simulink library "Ampere_Library"  (R2022b)
settings: Solver=FixedStepDiscrete  StartTime=0  StopTime=10.0  RelTol=1e-3  EnableMultiTasking=on
undefined symbols (not defined in the file or in its folder): A_INST_double, Dem_EventStatusType, ECU_AMBIENT_TEMPERATURE, SET_ECU_AMBIENT_TEMPERATURE, SlDemoSign, Std_ReturnType
libraries: simulink x13
(part 4 of 10)

== system Ampere_Library/User_Defined_Libraries/Logic_and_Bit_Operations ==
  note: Comparisons to value
  note: Detect changes for
      | booleans
  note: Detect changes for
      | all data types
  note: Logic & Bit Operations
  A_CompareToConstant : Subsystem  Tag=[LIB]  mask(A_CompareToConstant){relop===, Const=1, ZeroCross=off}
      mask prompts: relop "Operator:"; Const "Constant value:"; ZeroCross "Enable zero-crossing detection"
      mask help:
      | Output will be one when the signal less than or equal to a constant otherwise it will be zero.
      |
      | The "Operator" parameter can have the following values:
      |       1. "==" - Determine whether the input is equal to Constant.
      |       2. "~=" - Determine whether the input is not equal to Constant.
      |       3. "<"  - Determine whether the input is less than Constant.
      |       4. "<=" - Determine whether the input is less than or equal to Constant.
      |       5. ">"  - Determine whether the input is greater than Constant.
      |       6. ">=" - Determine whether the input is greater than or equal to Constant.
      |
      | Note:
      |       1. Input Datatype of the block must NOT be "Double" and "Single" when "==" or "~="  is used
      mask init:
      | %% Update internal relop block
      | set_param ([gcb,'/Compare'],'relop',relop, ...
      |     'ZeroCross', ZeroCross);
      settings: AttributesFormatString=%<MaskType>
      mask TypeOptions relop: == | ~= | < | <= | >= | >
      mask Callback ZeroCross:
      | % Update tag depending on the mask option Enable zero-crossing detection
      | if strcmp(get_param(gcb,'ZeroCross'),'on')
      |     % Display the SaturateOnOverflow parameter
      |     set_param(gcb, 'AttributesFormatString', sprintf('%%<MaskType>\nzero-crossing = on'));
      | else
      |     % Do not display the SaturateOnOverflow parameter
      |     set_param(gcb, 'AttributesFormatString', sprintf('%%<MaskType>\n'));
      | end
      mask Display:
      | %% Display info on the icon
      | fprintf('%s %s',relop, get(gcbh,'Const'));
  A_CompareToZero : Subsystem  Tag=[LIB]  mask(A_CompareToZero){relop===, ZeroCross=off}
      mask prompts: relop "Operator:"; ZeroCross "Enable zero-crossing detection"
      mask help:
      | A_CompareToZero block compares an input signal to zero.
      | Specify how the input is compared to zero with the "Operator" parameter.
      | The "Operator" parameter can have the following values:
      |       1. "==" - Determine whether the input is equal to zero.
      |       2. "~=" - Determine whether the input is not equal to zero.
      |       3. "<"  - Determine whether the input is less than zero.
      |       4. "<=" - Determine whether the input is less than or equal to zero.
      |       5. ">"  - Determine whether the input is greater than zero.
      |       6. ">=" - Determine whether the input is greater than or equal to zero.
      |
      | The output is 0 if the comparison is false, and 1 if it is true.
      |
      | Note:
      |       1. Input Datatype of the block must NOT be "Double" and "Single" when "==" or "~="  is used
      mask init:
      | %% Internal Parameter
      | cons_zero = 0;
      | 
      | %% Update Relop block properties
      | set_param([gcb,'/Compare'],'relop',relop, ...
      |     'ZeroCross', ZeroCross);
      settings: AttributesFormatString=%<MaskType>
      mask TypeOptions relop: == | ~= | < | <= | >= | >
      mask Callback ZeroCross:
      | if strcmp(get_param(gcb,'ZeroCross'),'on')
      |     % Display the SaturateOnOverflow parameter
      |     set_param(gcb, 'AttributesFormatString', sprintf('%%<MaskType>\nzero-crossing = on'));
      | else
      |     % Do not display the SaturateOnOverflow parameter
      |     set_param(gcb, 'AttributesFormatString', sprintf('%%<MaskType>\n'));
      | end
      mask Display:
      | %% Display info on the icon
      | fprintf('%s 0',relop);
  A_DEDGE : Subsystem  Tag=[LIB]  mask(A_DEDGE){}
      mask help:
      | Falling edge
      |
      | The output indicates true if the input value changes from true to false.
      |
      | Note:
      | The input of the block shall be a Boolean
      settings: AttributesFormatString=%<MaskType>
      mask Display:
      | %% Drawing the falling edge
      | plot([.5-0.2,.5,.5,.5+.2],[.5+.2,.5+.2,.5-.2,.5-.2]);
      | plot([.5-.05,.5,.5+.05],[.5+.05,.5-.05,.5+.05]);
  A_DetectChange : Subsystem  Tag=[LIB]  Variant=on  VariantControlMode=label  LabelModeActiveChoice=NonFloat_CompInit  mask(A_DetectChange){InputDataTyp=Non-Float, chkini=on, vinit=0, user_tol=eps}
      mask prompts: InputDataTyp "Input DataType"; chkini "Compare Input with Initial Value"; vinit "Initial Condition"; user_tol "Tolerance"
      mask help:
      | This block outputs TRUE when the input is not equal to its previous value.
      |
      | The "Input DataType" shall be selected as "Float" for floating data (Single / Double) or "Non-Float" otherwise (Boolean / Integer / Enum / Fixdt).
      |
      | The "Initial Condition" can be specified by ticking the "Compare Input with Initial Value" option and determines the initial value of the previous input U/z.
      | If this option is unticked, the block outputs FALSE at its first execution.
      |
      | When "Input DataType" is selected as "Float", the user defines the tolerance used to do the comparison which shall not be 0.
      | For floating data, the comparison is done with the following algorithm: abs(U-U/z)>tolerance.
      |
      | Specific use case : When using this block with a signal having an enumerated data type and with "Compare Input with Initial Value" unticked,  the "Initial Condition" has to be specified anyway even if it is unused. In this use case, the user first ticks the "Compare Input with Initial Value" option, and fills the "Initial Condition" field with a valid enumerated value of the desired data type (ex: the native SlDemoSign enumeration has a value SlDemoSign.Negative). Then the user unticks "Compare Input with Initial Value", and can use the block.
      mask init:
      | %% Get values for the option chosen by the user
      | CompInit = strcmp(get(gcbh,'chkini'),'on');
      | Flt = strcmp(get(gcbh,'InputDataTyp'),'Float');
      | 
      | %% Setting the tolerance in case of floating data
      | if Flt
      |     % If the tolerance is 0, it is reset to eps and an error dialog box
      |     % informs the user.
      |     if user_tol == 0
      |         errordlg(sprintf(['"0" Tolerance is not allowed.\n',...
      |             'The parameter %s is replaced with "eps" in the block\n%s'],...
      |             get(gcbh,'user_tol'),regexprep(gcb,'\n','')),...
      |             'A_DetectChange');
      |         set(gcbh,'user_tol','eps');
      |         user_tol = eps;
      |     end
      |     tol = user_tol;
      | end
      | 
      | %% Change the attributesFormatString depending of the different combination
      | % of the options, and define the active variant (variable "selection").
      | if  Flt && CompInit
      |     % Case Float + Init Compare
      |     selection = 'Float_CompInit';
      |     set(gcbh,'AttributesFormatString',sprintf('%%<MaskType>\nIC = %%<vinit>\nTol = %%<user_tol>'));
      | 
      | elseif Flt && ~CompInit
      |     % Case Float + No Init Compare
      |     selection = 'Float_NoComp';
      |     set(gcbh,'AttributesFormatString',sprintf('%%<MaskType>\nTol = %%<user_tol>'));
      | 
      | elseif ~Flt && CompInit
      |     % Case Non-Float + Init Compare
      |     selection = 'NonFloat_CompInit';
      |     set(gcbh,'AttributesFormatString',sprintf('%%<MaskType>\nIC = %%<vinit>'));
      |     % Reset the user tolerance in case of Non-Float to avoid keeping
      |     % unused variable name in the block.
      |     set(gcbh,'user_tol','eps');
      |     
      | else
      |     % else case : ~Flt && ~CompInit
      |     % Case Non-Float + No Init Compare
      |     selection = 'NonFloat_NoComp';
      |     set(gcbh,'AttributesFormatString',sprintf('%%<MaskType>'));
      |     % Reset the user tolerance in case of Non-Float to avoid keeping
      |     % unused variable name in the block.
      |     set(gcbh,'user_tol','eps');
      | end
      | 
      | %% Change the active Variant according to the user's choices.
      | set(gcbh,'OverrideUsingVariant',selection);
      settings: AttributesFormatString=|
      | %<MaskType>
      | IC = %<vinit>
      mask TypeOptions InputDataTyp: Float | Non-Float
      mask Callback InputDataTyp:
      | %% Makes "Tolerance" visible depending on the "Float" option
      | Maskvisibilities = get(gcbh,'Maskvisibilities');
      | if strcmp(get(gcbh,'InputDataTyp'),'Float')
      |     Maskvisibilities{4} = 'on';
      | else
      |     Maskvisibilities{4} = 'off';
      | end
      | set(gcbh,'Maskvisibilities',Maskvisibilities);
      mask Callback chkini:
      | %% Makes "Init Value" visible depending on the "Compare Init" option
      | Maskvisibilities = get(gcbh,'Maskvisibilities');
      | if strcmp(get(gcbh,'chkini'),'on')
      |     Maskvisibilities{3} = 'on';
      | else
      |     Maskvisibilities{3} = 'off';
      | end
      | set(gcbh,'Maskvisibilities',Maskvisibilities);
      mask Display:
      | %% Display infos on the mask
      | fprintf('U ~= U/z\n%s',get(gcbh,'InputDataTyp'));
  A_DetectIncDec : Subsystem  Tag=[LIB]  mask(A_DetectIncDec){Detect_chg=Detect Decrease, chkini=on, vinit=0}
      mask prompts: Detect_chg "Detect Change Input"; chkini "Compare the Input with Initial Value"; vinit "Initial Value"
      mask help:
      | Detect Decrease:
      | If the input is strictly lesser than its previous value, then output TRUE, otherwise output FALSE. Initial condition of the output is false.
      | Detect Increase:
      | If the input is strictly greater than its previous value, then output TRUE, otherwise output FALSE. Initial condition of the output is false.
      |
      | NOTE:
      | The check for the initial condidtion can be inhibited by unchecking the checkbox
      | "Compare the Input with Initial Value".
      mask init:
      | %% Update internal Relop block for Increase or Decrease case
      | switch Detect_chg
      |     case 1
      |         % Increase
      |         set_param([gcb '/IncDec'],'Operator','>');
      |     case 2
      |         % Decrease
      |         set_param([gcb '/IncDec'],'Operator','<');
      | end
      | 
      | %% Update internal "From" block depending of the "Compare Input with Initial Value" option
      | if strcmp(get_param(gcb,'chkini'),'on')
      |     set_param([gcb '/From'],'GotoTag','fromRelOpe');
      | else
      |     set_param([gcb '/From'],'GotoTag','vchk_val');
      | end
      settings: AttributesFormatString=|
      | %<MaskType>
      | IC = %<vinit>
      mask TypeOptions Detect_chg: Detect Increase | Detect Decrease
      mask Callback chkini:
      | %% Make the "Compare Input with Initial Value" visible or not in the mask
      | if strcmp(get_param(gcb,'chkini'),'on')
      |     set_param(gcb,'Maskvisibilities',{'on','on','on'});
      |     set_param(gcb,'AttributesFormatString',sprintf('%%<MaskType>\nIC = %%<vinit>'));
      | else
      |     set_param(gcb,'Maskvisibilities',{'on','on','off'});
      |     set_param(gcb,'AttributesFormatString','%<MaskType>');
      | end
      mask Display:
      | %% Display the Icon depending of the option
      | if Detect_chg==1
      |     % Case Increase
      |     fprintf('U > U/z')
      | else
      |     % Case Decrease
      |     fprintf('U < U/z')
      | end
  A_EdgeDetect_Ext_IC : Subsystem  Tag=[LIB]  mask(A_EdgeDetect_Ext_IC){Edge_type=Rising, chkini=off, InitOut=false}
      mask prompts: Edge_type "Hit crossing direction"; chkini "Compare the Input with Initial Value"; InitOut "Initial Output :"
      mask help:
      | This block can be used to :
      | 	* Detect change
      | 	* Detect increase
      | 	* Detect decrease
      |
      | If "Compare the Input with Initial Value" is checked, at the first time-step, the output depends on the comparison between "In" and "IC".
      | Otherwise, the output at the first time step is set by the parameter 'Initial Output'.
      | The output is a signal of data type 'boolean'.
      |
      | Note : Both inputs should be "boolean" DataType.
      mask init:
      | %% Common parameters for plotting the icon
      | a = 0.3;
      | b = 0.5;
      | c = 0.7;
      | 
      | %% Update From block and parameter for icon display
      | if Edge_type == 1
      |     % Rising
      |     set_param([gcb '/VarSelect'], 'GotoTag', 'RisingEdge');
      |     d = 0.6;
      |     e = 0.9;
      |     f = 0.6;
      |     g = 0.9;
      | 
      | elseif Edge_type == 2
      |     % Falling
      |     set_param([gcb '/VarSelect'], 'GotoTag', 'FallingEdge');
      |     d = 0.9;
      |     e = 0.6;
      |     f = 0.9;
      |     g = 0.6;
      | 
      | else
      |     % Either
      |     set_param([gcb '/VarSelect'], 'GotoTag', 'Either');
      |     d = 0.9;
      |     e = 0.6;
      |     f = 0.6;
      |     g = 0.9;
      | end
      | 
      | %% Create the infos to display below the block depending of the Mask Options
      | % Always display MaskType
      | Attrib = '%<MaskType>\nCompInit = %<chkini>';
      | % Conditionnally adding Initial value
      | if strcmp(get_param(gcb,'chkini'),'off')
      |     Attrib = [Attrib '\nIC =  %<InitOut>'];
      | end
      | % Update the display
      | set_param(gcb,'AttributesFormatString',Attrib);
      settings: AttributesFormatString="%<MaskType>\\nCompInit = %<chkini>\\nIC =  %<InitOut>"
      mask TypeOptions Edge_type: Rising | Falling | Either
      mask Callback chkini:
      | %% Update tag depending on the mask option Compare Input with Initial Value
      | if strcmp(get_param(gcb,'chkini'),'on')
      |     set_param(gcb,'Maskvisibilities',{'on','on','off'});
      |     set_param([gcb '/From'],'GotoTag','Check_Type');
      | else
      |     set_param(gcb,'Maskvisibilities',{'on','on','on'});
      |     set_param([gcb '/From'],'GotoTag','vchk_val')
      | end
      mask TypeOptions InitOut: false | true
      mask Callback InitOut:
      | %% Update Constant value depending on the mask option Initial Output
      | if strcmp(get_param(gcb,'InitOut'),'false')
      |     set_param([gcb '/InitOutVal'],'value','false');
      | else
      |     set_param([gcb '/InitOutVal'],'value','true');
      | end
      mask Display:
      | %% Plot the different edges
      | % green only visible in case Either, and plot "Rising"
      | color('green');
      | plot([a b b c],[f f g g]);
      | 
      | % Rising or Falling when selected, or Falling in case Either
      | color('red');
      | plot([a b b c],[d d e e]);
      | 
      | % Impulse triggering the edge
      | color('blue');
      | plot([a b b b c],[0.1 0.1 0.4 0.1 0.1]);
  A_Either_EdgeDetect : Subsystem  Tag=[LIB]  mask(A_Either_EdgeDetect){}
      mask help:
      | Either edge
      |
      | The output indicates true at any change of the logical input value
      |
      | Note:
      | The input of the block shall be a Boolean
      settings: AttributesFormatString=%<MaskType>
      mask Display:
      | %% Drawing the rising and falling edges
      | plot([.5-0.2,.5,.5,.5+.2],[.5-.25,.5-.25,.5+.25,.5+.25]);
      | plot([.5-.05,.5,.5+.05],[.59-.05,.59+.05,.59-.05]);
      | plot([.5-.05,.5,.5+.05],[.41+.05,.41-.05,.41+.05]);
  A_UEDGE : Subsystem  Tag=[LIB]  mask(A_UEDGE){}
      mask help:
      | Rising edge
      |
      | The output indicates true if the input value changes from false to true.
      |
      | Note :
      | The input of the block shall be a Boolean
      settings: AttributesFormatString=%<MaskType>
      mask Display:
      | %% Drawing the rising edge
      | plot([.5-0.2,.5,.5,.5+.2],[.5-.2,.5-.2,.5+.2,.5+.2]);
      | plot([.5-.05,.5,.5+.05],[.5-.05,.5+.05,.5-.05]);

== system Ampere_Library/User_Defined_Libraries/Lookup_Tables ==
  note: Other
  note: Cos and sin for fixdt
      | using lookup tables
  note: Obsolete
  note: Lookup Tables
  A_Carto1D : Subsystem  Tag=[LIB]  mask(A_Carto1D){x=[1 2 3 4 5 ], z=[10 20 30 40 50], SaturateOnOverflow=off}
      mask prompts: x "Breakpoint table :"; z "Cartography table :"; SaturateOnOverflow "Saturate on integer overflow"
      mask help:
      | ***********************************
      | OBSOLETE
      | Use native "One_D_Lookup_Table" block available in MBD_Base_Blocks/Simulink/Lookup_Tables
      | ***********************************
      |
      |
      | This block executes an interpolation in a one-dimension cartography.
      |
      | Use the Mask Parameters to provide Break point and Lookup Tables.
      mask init:
      | %% If the user don't specify x or z, then default atan definition is used
      | % this use case should not occur in real projects.
      | if isempty(x)||isempty(z)
      |     fprintf(2,'The bloc %s is missing x or z data\n',gcb);
      |     x = -5:0.5:5;
      |     z = atan(-5:0.5:5);
      | end
      settings: AttributesFormatString=|
      | %<MaskType>
      | Breakpoint table = %<x>
      | Cartography table = %<z>
      | SAT = %<SaturateOnOverflow>
      mask TypeOptions SaturateOnOverflow: data_1D_Lookup_Table/SaturateOnIntegerOverflow
      mask Display:
      | %% Display the text in top middle
      | text(.5,.8,'A Carto1D','HorizontalAlignment','center');
  A_Carto2D : Subsystem  Tag=[LIB]  mask(A_Carto2D){map_x=[ -214748364.8 0 ], map_y=[ -214748364.8 -1 ], carto=[ -214748364.8 35; 249 64 ; ], SaturateOnOverflow=off}
      mask prompts: map_x "X breakpoint table :"; map_y "Y breakpoint table :"; carto "cartography name :"; SaturateOnOverflow "Saturate on integer overflow for LookUp table"
      mask help:
      | ***********************************
      | OBSOLETE
      | Use native "Two_D_Lookup_Table" block available in MBD_Base_Blocks/Simulink/Lookup_Tables
      | ***********************************
      |
      |
      | This block executes an interpolation in a two-dimension cartography.
      settings: AttributesFormatString=|
      | %<MaskType>\nX breakpoint table = %<map_x>\nY breakpoint table = %<map_y>\ncartography name = %<carto>
      | SAT = %<SaturateOnOverflow>
      mask TypeOptions SaturateOnOverflow: LookupTable2D/SaturateOnIntegerOverflow
      mask Display:
      | %% Display the text in top middle
      | text(0.5,0.85,'A Carto2D','HorizontalAlignment','center');
  A_Cosine : Subsystem  Tag=[LIB]  mask(A_Cosine){NumDataPoints=32, OutputWordLength=8, FractionDataTypeStr=double}
      mask prompts: NumDataPoints "Number of data points for Lookup table:"; OutputWordLength "Output Word Length:"; FractionDataTypeStr "Simulink:blkprm_prompts:LookupNdFractionUnifType"
      mask help: The block implements a Cosine wave in fixed point using lookup table method that is based on quarter wave symmetry.
      mask init:
      | %% Internal parameters
      | Cons_P25 = 0.25;
      | Cons_P5 = 0.5;
      | Cons_P75 = 0.75;
      | Cons_M1 = -1;
      | 
      | %% Compute Table for LUT
      | k = linspace(0,0.25,NumDataPoints);
      | b = zeros(1,NumDataPoints);
      | for i = 1:NumDataPoints
      |     l = 0;
      |     for j = 1:2:63
      |         l = l+1;
      |         if rem(l,2)
      |             b(i) = b(i) + (power(k(i)*2*pi,j)/factorial(j));
      |         else
      |             b(i) = b(i) - (power(k(i)*2*pi,j)/factorial(j));
      |         end
      |     end
      | end
      | 
      | %% Compute OutputFracLength
      | OutputFracLength = OutputWordLength-2;
      settings: AttributesFormatString=%<MaskType>\nLUT Nb points = %<NumDataPoints>\nWord Length = %<OutputWordLength>
      mask TypeOptions FractionDataTypeStr: LookupTable1_D/FractionDataTypeStr
      mask DialogControl FractionDataTypeStr Prompt: Fraction data type:
      mask Display:
      | %% Display info on the icon
      | fprintf('cos(x)\nfixdt')
  A_LookupTableDynamic : Subsystem  Tag=[LIB]  mask(A_LookupTableDynamic){tolerance=Absolute Zero, user_tol=10, SaturateOnIntegerOverflow=off}
      mask prompts: tolerance "Tolerance for Division"; user_tol "User Tolerance"; SaturateOnIntegerOverflow "Simulink:blkprm_prompts:AllBlksSaturate"
      mask help:
      | ***********************************
      | OBSOLETE
      | Use native "LookupTableDynamic" block available in MBD_Base_Blocks/Simulink/Lookup_Tables, configured as "Use Input Below" for equivalence to this block.
      | ***********************************
      |
      | The Lookup Table Dynamic block computes an approximation of a function y = f(x) using xdat and ydat vectors. The lookup method can use interpolation or the original values of the input.
      | Using the Lookup Table Dynamic block, the table data can be changed without stopping the simulation.
      |
      | The Values for xdat should be strictly monotonical increasing order.
      |
      | The rounding method 'zero' is used for all arithmetic calculations.
      mask init:
      | %% Internal parameters
      | cons1 = 1;
      | cons0 = 0;
      | divchk = 0;
      | 
      | %% Compute tolerance
      | switch tolerance
      |    case 1
      |        divchk = eps('double');
      |    case 2
      |        divchk = eps('single');
      |    case 3
      |        divchk = 0;
      |    case 4
      |        divchk = user_tol;
      | end
      | 
      | %% Create the infos to display below the block depending of the Mask Options
      | % Always display MaskType
      | Attrib = '%<MaskType>';
      | % Conditionnally adding Tolerance value
      | if strcmp(get_param(gcb,'tolerance'),'User Defined')
      |     Attrib = [Attrib '\nTolerance = %<user_tol>'];
      | end
      | % Conditionnally adding Saturation
      | if strcmp(get_param(gcb,'SaturateOnIntegerOverflow'),'on')
      |     Attrib = [Attrib '\nSAT = on'];
      | end
      | % Update the display
      | set_param(gcb,'AttributesFormatString',Attrib);
      settings: AttributesFormatString=%<MaskType>
      mask TypeOptions tolerance: eps Double | eps Single | Absolute Zero | User Defined
      mask Callback tolerance:
      | %% Make visible or not the Tolerance Value (update 2nd element of MaskVisibilities)
      | MaskVisibilities = get_param(gcb,'MaskVisibilities');
      | if strcmp(get_param(gcb,'tolerance'),'User Defined')
      |     MaskVisibilities{2} = 'on';
      | else
      |     MaskVisibilities{2} = 'off';
      | end
      | set_param(gcb,'MaskVisibilities',MaskVisibilities);
      mask TypeOptions SaturateOnIntegerOverflow: Divide/SaturateOnIntegerOverflow | Product1/SaturateOnIntegerOverflow | Product2/SaturateOnIntegerOverflow | Sum1/SaturateOnIntegerOverflow | Sum2/SaturateOnIntegerOverflow | Sum3/SaturateOnIntegerOverflow | Sum5/SaturateOnIntegerOverflow | Sum6/SaturateOnIntegerOverflow | Sum7/SaturateOnIntegerOverflow | Switch/SaturateOnIntegerOverflow | Switch1/SaturateOnIntegerOverflow | Switch3/SaturateOnIntegerOverflow | Switch4/SaturateOnIntegerOverflow | Switch5/SaturateOnIntegerOverflow | Switch6/SaturateOnIntegerOverflow
      mask DialogControl SaturateOnIntegerOverflow Prompt: Saturate on integer overflow
  A_SaturatedLookUpTable : Subsystem  Tag=[LIB]  mask(A_SaturatedLookUpTable){input_vector=single([-5;5]), output_vector=single(tanh([-5;5])), TableResolution=single(0.1), lup_mthd=Interpolation - Use End Values, prod_OutDataTypeStr=single}
      mask prompts: input_vector "BreakPoint Table"; output_vector "Lookup Table"; TableResolution "Resolution of output signal"; lup_mthd "LookUp Method"; prod_OutDataTypeStr "Simulink:blkprm_prompts:OUTPUT_UNIFIEDDATATYPE"
      mask help:
      | This block Performs 1-D Linear/Flat interpolation.
      | Initially the Input signal 'in' is limited between two extreme values of the breakpoint table, then it is converted to the specific resolution as defined in the mask parameter "Resolution of output signal"to obtain the output "Out". Thus extrapolation is not performed outside of the table boundaries.
      |
      | Interpolation Method can be selected as required either to "Linear(Use End Values)" or "Flat (Use Input Below)".
      |
      | When the mask parameter "LookUp Method" is chosen as "Use End value", it performs 1D lookup table operation with linear interpolation and convert this data to a specified resolution.
      |
      | When the mask parameter "LookUp Method" is chosen as "Use Input value", it performs 1D lookup table operation with flat interpolation and convert this data to a specified resolution.
      |
      |
      | Note :
      | 1. This block will work upto the range of UINT32 MAX which means Absolute value of Input should NOT exceed beyond UINT32 MAX.
      | 2. Resolution should not be ZERO. If Zero provided, implicitly block will consider it as ONE.
      | 3. Output data type of the block has to be chosen by the user through "Output data type" mask parameter.
      mask init:
      | %% Internal parameters
      | RF0 = single(0);
      | RF5 = single(0.5);
      | RF1 = single(1);
      | 
      | %% LookUp Method
      | switch lup_mthd
      |     case 1
      |         set_param([gcb '/OneD_Lookup_Table'],'InterpMethod','Linear');
      |     case 2
      |         set_param([gcb '/OneD_Lookup_Table'],'InterpMethod','Flat');
      | end
      | 
      | %% Resolution of output signal
      | if TableResolution == 0
      |     Resolution = 1;
      | else
      |     Resolution = TableResolution;
      | end
      settings: AttributesFormatString=%<MaskType>
      mask TypeOptions lup_mthd: Interpolation - Use End Values | Use Input Below
      mask TypeOptions prod_OutDataTypeStr: Product1/OutDataTypeStr
      mask DialogControl prod_OutDataTypeStr Prompt: Output data type:
      mask Display:
      | %% Display parameters values
      | fprintf('BK = %s\nLUT = %s', get_param(gcb,'input_vector'), get_param(gcb,'output_vector'));
  A_Sine : Subsystem  Tag=[LIB]  mask(A_Sine){NumDataPoints=32, OutputWordLength=8, FractionDataTypeStr=double}
      mask prompts: NumDataPoints "Number of data points for lookup table:"; OutputWordLength "Output word length:"; FractionDataTypeStr "Simulink:blkprm_prompts:LookupNdFractionUnifType"
      mask help: Implements a sine wave in fixed point using a lookup table method that which is based on quarter wave symmetry.
      mask init:
      | %% Internal parameters
      | Cons_P25 = 0.25;
      | Cons_P5 = 0.5;
      | Cons_M1 = -1;
      | 
      | %% Compute Table for LUT
      | k = linspace(0,0.25,NumDataPoints);
      | b = zeros(1,NumDataPoints);
      | for i = 1:NumDataPoints
      |     l = 0;
      |     for j = 1:2:63
      |         l = l+1;
      |         if rem(l,2)
      |             b(i) = b(i) + (power(k(i)*2*pi,j)/factorial(j));
      |         else
      |             b(i) = b(i) - (power(k(i)*2*pi,j)/factorial(j));
      |         end
      |     end
      | end
      | 
      | %% Compute OutputFracLength
      | OutputFracLength = OutputWordLength-2;
      settings: AttributesFormatString=%<MaskType>\nLUT Nb points = %<NumDataPoints>\nWord Length = %<OutputWordLength>
      mask TypeOptions FractionDataTypeStr: LookupTable1_D/FractionDataTypeStr
      mask DialogControl FractionDataTypeStr Prompt: Fraction data type:
      mask Display:
      | %% Display info on the icon
      | fprintf('sin(x)\nfixdt')

== system Ampere_Library/User_Defined_Libraries/Math_Operations ==
  note: Rounding and modulo
  note: Protected divisions
  note: Powers
  note: Math Operations
  A_ADivB : Subsystem  Tag=[LIB]  mask(A_ADivB){divbyzval=0, Den_Tol=Absolute Zero tol, user_tol=0, SaturateOnOverflow=off, prod_OutDataTypeStr=Inherit: Inherit via back propagation}
      mask prompts: divbyzval "Control Value if Den <= Tolerance"; Den_Tol "Tolerance"; user_tol "User Defined Tolerance"; SaturateOnOverflow "Saturate on integer overflow"; prod_OutDataTypeStr "Simulink:blkprm_prompts:OUTPUT_UNIFIEDDATATYPE"
      mask help:
      | This block gives output of "AdivB" by dividing two inputs "A" and "B".
      | If Absolute value of B is less than or equal to Tolerance, output will be "A" Divided by "Control Value".
      |
      | Note: Output data type of the block has to be chosen by the user through "Output data type" mask parameter.
      mask init:
      | %% Compute the tolerance
      | switch Den_Tol
      |     case 1
      |         tol = eps('double');
      |     case 2
      |         tol = eps('single');
      |     case 3
      |         tol = 0;
      |     case 4
      |         tol = user_tol;
      | end
      | 
      | %% Create the infos to display below the block depending of the Mask Options
      | % Always display MaskType
      | Attrib = '%<MaskType>\nCtrl Val = %<divbyzval>';
      | % Conditionnally adding Tolerance
      | if strcmp(get_param(gcb,'Den_Tol'),'User Defined tol')
      |     Attrib = [Attrib '\nTol = %<user_tol>'];
      | end
      | % Conditionnally adding Sat
      | if strcmp(get_param(gcb,'SaturateOnOverflow'),'on')
      |     Attrib = [Attrib '\nSAT = on'];
      | end
      | % Update the display
      | set_param(gcb,'AttributesFormatString',Attrib);
      settings: AttributesFormatString=%<MaskType>\nCtrl Val = %<divbyzval>
      mask TypeOptions Den_Tol: double tol - eps('double') | single tol - eps('single') | Absolute Zero tol | User Defined tol
      mask Callback Den_Tol:
      | %% Make visible or not the Tolerance (update 3rd element of MaskVisibilities)
      | MaskVisibilities = get_param(gcb,'MaskVisibilities');
      | if strcmp(get_param(gcb,'Den_Tol'),'User Defined tol')
      |     MaskVisibilities{3} = 'on';
      | else
      |     MaskVisibilities{3} = 'off';
      | end
      | set_param(gcb,'MaskVisibilities',MaskVisibilities);
      mask TypeOptions SaturateOnOverflow: Switch/SaturateOnIntegerOverflow | Divide/SaturateOnIntegerOverflow | Abs1/SaturateOnIntegerOverflow
      mask TypeOptions prod_OutDataTypeStr: Divide/OutDataTypeStr
      mask DialogControl prod_OutDataTypeStr Prompt: Output data type:
  A_DivisionByZero : Subsystem  Tag=[LIB]  mask(A_DivisionByZero){Den_Tol=0, SaturateOnOverflow=off}
      mask prompts: Den_Tol "Denominator Tolerance"; SaturateOnOverflow "Saturate on Integer Overflow"
      mask help: This block outputs the value of the division operation "num / den ". If the "den" is less than "Denominator Tolerance", the output will be the value at the port "default".
      settings: AttributesFormatString=%<MaskType>\nTol = %<Den_Tol>
      mask TypeOptions SaturateOnOverflow: Abs1/SaturateOnIntegerOverflow | Divide/SaturateOnIntegerOverflow | Switch/SaturateOnIntegerOverflow
      mask Callback SaturateOnOverflow:
      | %% Create the infos to display below the block depending of the Mask Options
      | % Default Parameters Display
      | Attrib = '%<MaskType>\nTol = %<Den_Tol>';
      | % Add conditional display of saturation
      | if strcmp(get_param(gcb,'SaturateOnOverflow'),'on')
      |     Attrib = [Attrib '\nSAT = on'];
      | end
      | % Update Attributes Display
      | set_param(gcb, 'AttributesFormatString', (Attrib));
      mask Display:
      | %% Display info on the icon
      | fprintf('Division\nno div by "0"')
  A_Modulo : Subsystem  Tag=[LIB]  mask(A_Modulo){InternalDataType=uint16, Den=Double Tol, User_Value=0, chkdt=on, SaturateOnOverflow=off}
      mask prompts: InternalDataType "Data Type for output of Division"; Den "Tolerance For Floating Point Comparison To Zero"; User_Value "User Defined Tolerance Value"; chkdt "Input of Unsigned Datatype"; SaturateOnOverflow "Saturate on integer overflow"
      mask help:
      | Description
      | M = mod(X,Y) returns the modulus after division of X by Y.
      |
      | If Y does not equal 0, M = mod(X,Y) returns X - n.*Y, where n = floor(X./Y)
      | Inputs X and Y must have the same dimensions unless one is a scalar double.
      | If one input has an integer data type, then the other input must be of the same integer data type or be a scalar double.
      |
      | <Data Type For Internal Calculations> parameter defines possible data types for the operation x./y
      | Tune this parameter as per max and min possible values of x and y;
      |  - If uint8 is selected, the block calculates correct results up to the value of the ratio x./y is <= intmax('uint8');
      |  - If uint16 is selected, the block calculates correct results up to the value of the ratio x./y is <= intmax('uint16');
      |  - If uint32 is selected, the block calculates correct results up to the value of the ratio x./y is <= intmax('uint32');
      |
      | <Tolerance For Floating Point Comparison To Zero> : Tune this parameter as follows :
      |   - Select <Double Tol> if block's inputs are of Double data type (eps('double'))
      |   - Select <Single Tol > if block's inputs are of Single data type (eps('single'))
      |   - Select <Absolute Zero Tol> if block's inputs are of Integer of fixdt datatype (0)
      |   - Select <User Defined Tol> to define custom tolerance value.
      | If the selected value is <User Defined Tol> the parameters <User Division Tolerance Value> and <User Value DataType> are enabled. The data type must be the same as block's inputs data type, select <Inherit : ....> to inherit this data type from block's inputs if defined.
      | An error occurs if tolerance selection is not performed as specified above.
      | An error occurs if inputs are not of the same data type.
      |
      | Note:
      | 1)The two inputs x and y must have the same data type.
      | 2)The result of Abs(X)/Abs(Y) should not exceed the Maximum value of the data type selected in "<Data Type For Internal Calculations>"
      | 3)For inputs with signed data type, Minimum value of the signed data type should not be passed as input.
      | 4)For RTW code generation select "Remove code that protects against division arithmetic exceptions" option in Configuration Parameters settings.
      |
      | The following are true by convention:
      | - mod(X,0) is X
      | - mod(X,X) is 0
      | - mod(X,Y) for X~=Y and Y~=0 has the same sign as Y
      mask init:
      | %% Internal parameters
      | cmpTol = 0;
      | cmpZero = 0;
      | cste0 = 0;
      | constOne = 1;
      | 
      | %% Update internal From tag
      | if strcmp(get_param(gcb,'chkdt'),'on')
      |     set_param([gcb '/From19'],'GotoTag','constone');
      | else
      |     set_param([gcb '/From19'],'GotoTag','Mulconst');
      | end
      | 
      | %% Compute the tolerance
      | switch Den
      |     case 'Double Tol'
      |         cmpTol = eps('double');
      |     case 'Single Tol'
      |         cmpTol = eps('single');
      |     case 'Absolute Zero Tol'
      |         cmpTol = 0;
      |     case'User Defined Tol'
      |         cmpTol = User_Value;
      | end
      | 
      | %% Create the infos to display below the block depending of the Mask Options
      | % Always display MaskType
      | Attrib = '%<MaskType>';
      | % Conditionnally adding Tolerance
      | if strcmp(get_param(gcb,'Den'),'User Defined Tol')
      |     Attrib = [Attrib '\nTol = %<User_Value>'];
      | end
      | % Conditionnally adding Sat
      | if strcmp(get_param(gcb,'SaturateOnOverflow'),'on')
      |     Attrib = [Attrib '\nSAT = on'];
      | end
      | % Update the display
      | set_param(gcb,'AttributesFormatString',Attrib);
      settings: AttributesFormatString=%<MaskType>
      mask TypeOptions Den: Double Tol | Single Tol | Absolute Zero Tol | User Defined Tol
      mask Callback Den:
      | %% Make visible or not the Tolerance (update 3rd element of MaskVisibilities)
      | MaskVisibilities = get_param(gcb,'MaskVisibilities');
      | if strcmp(get_param(gcb,'Den'),'User Defined Tol')
      |     MaskVisibilities{3} = 'on';
      | else
      |     MaskVisibilities{3} = 'off';
      | end
      | set_param(gcb,'MaskVisibilities',MaskVisibilities);
      mask TypeOptions SaturateOnOverflow: Abs1/SaturateOnIntegerOverflow | Abs2/SaturateOnIntegerOverflow | Add1/SaturateOnIntegerOverflow | Add2/SaturateOnIntegerOverflow | Product1/SaturateOnIntegerOverflow | Product2/SaturateOnIntegerOverflow | Switch/SaturateOnIntegerOverflow | Switch4/SaturateOnIntegerOverflow
      mask Display: fprintf('M = mod(X,Y)\nUnsigned = %s',get_param(gcbh,'chkdt'));
  A_RoundingFunction : Subsystem  Tag=[LIB]  mask(A_RoundingFunction){mini_val=double tol - eps('double'), user_tol=0, Rounding_function=Round}
      mask prompts: mini_val "Tolerance for internal calculation"; user_tol "User Defined Tolerance"; Rounding_function "Function"
      mask help:
      | The Rounding Function block performs a round operation to the input signal as per the round method selected in the mask parameter. User can select one of the following rounding functions from the Function list:
      | 1. Floor
      | 2. Ceil
      | 3. Round
      | 4. Nearest
      | 5. Fix
      |
      | Choose the "Tolerance for internal calculation" as below.
      |
      | 1.Default option is 'double tol - eps(''double'')', which is for  double datatype.
      | 2.For single datatype, it is 'single tol - eps('single')
      | 3.For zero tolerance choose it as 'Absolute Zero tol'
      | 4.For specific value of tolerance, choose 'User Defined tol'
      | Specify "User Defined Tolerance" with the custom value required.
      mask init:
      | %% Internal parameters
      | Rounding_function = uint8(Rounding_function-1);
      | RF0 = 0;
      | RF1 = 1;
      | RF5 = 0.5;
      | 
      | %% Update From block to output the expected user choice
      | switch get_param(gcb, 'Rounding_function')
      |     case 'Floor'
      |         set_param([gcb '/VarFrom'], 'GotoTag', 'Floor_out');
      |     case 'Ceil'
      |         set_param([gcb '/VarFrom'], 'GotoTag', 'Ceil_out');        
      |     case 'Round'
      |         set_param([gcb '/VarFrom'], 'GotoTag', 'Round_out');        
      |     case 'Fix'
      |         set_param([gcb '/VarFrom'], 'GotoTag', 'Fix_out');        
      |     case 'Nearest'
      |         set_param([gcb '/VarFrom'], 'GotoTag', 'Near_out');   
      | end
      | 
      | %% Compute the tolerance
      | switch mini_val
      |    case 1
      |        tol = eps('double');
      |    case 2
      |        tol = eps('single');
      |    case 3
      |        tol = 0;
      |    case 4
      |        tol = user_tol;
      | end
      | 
      | %% Create the infos to display below the block depending of the Mask Options
      | % Always display MaskType
      | Attrib = '%<MaskType>';
      | % Conditionnally adding Tolerance
      | if strcmp(get_param(gcb,'mini_val'),'User Defined tol')
      |     Attrib = [Attrib '\nTol = %<user_tol>'];
      | end
      | % Update the display
      | set_param(gcb,'AttributesFormatString',Attrib);
      settings: AttributesFormatString=%<MaskType>
      mask TypeOptions mini_val: double tol - eps('double') | single tol - eps('single') | Absolute Zero tol | User Defined tol
      mask Callback mini_val:
      | %% Make visible or not the Tolerance (update 3rd element of MaskVisibilities)
      | MaskVisibilities = get_param(gcb,'MaskVisibilities');
      | if strcmp(get_param(gcb,'mini_val'),'User Defined tol')
      |     MaskVisibilities{2} = 'on';
      | else
      |     MaskVisibilities{2} = 'off';
      | end
      | set_param(gcb,'MaskVisibilities',MaskVisibilities);
      mask TypeOptions Rounding_function: Floor | Ceil | Round | Fix | Nearest
      mask Display:
      | %% Display info on the icon
      | fprintf('%s',get(gcbh,'Rounding_function'))
  A_SquareRoot : Subsystem  Tag=[LIB]  mask(A_SquareRoot){Tol=Absolute Zero Tol, User_Value=0, SATOnIntegerOverflow=off}
      mask prompts: Tol "Tolerance For Comparison To Zero"; User_Value "User Defined Tolerance Value"; SATOnIntegerOverflow "Simulink:blkprm_prompts:AllBlksSaturate"
      mask help:
      | This block provides the square root of the input signal as Output.
      |
      | <Tolerance For Comparison To Zero> : Tune this parameter as follows :
      |   - Select <Double Tol> if input is of Double data type (eps('double'))
      |   - Select <Single Tol > if input is of Single data type (eps('single'))
      |   - Select <Absolute Zero Tol> if input is of Integer of fixed point datatype.
      |   - Select <User Defined Tol> to define custom tolerance value.
      | Note:
      | 1) This block will give output as '0', when negative values are passed as input.
      | 2) This block will not support fixed point data type
      | 3) For inputs with double data type, block will support for the following range (0 to 3.4028e+38).
      mask init:
      | %% Internal Parameters
      | UdicVal = 64;
      | Cons2 = 2;
      | numofiter = 80;
      | constZero = 0;
      | 
      | %% Compute Tolerance
      | switch get_param(gcb,'Tol')
      |     case 'Double Tol'
      |         cmpTol = eps('double');
      |     case 'Single Tol'
      |         cmpTol = eps('single');
      |     case 'Absolute Zero Tol'
      |         cmpTol = 0;
      |     case 'User Defined Tol'
      |         cmpTol = User_Value;
      | end
      | 
      | %% Create the infos to display below the block depending of the Mask Options
      | % Always display MaskType
      | Attrib = '%<MaskType>';
      | % Conditionnally adding Tolerance
      | if strcmp(get_param(gcb,'Tol'),'User Defined Tol')
      |     Attrib = [Attrib '\nTol = %<User_Value>'];
      | end
      | % Conditionnally adding Sat
      | if strcmp(get_param(gcb,'SATOnIntegerOverflow'),'on')
      |     Attrib = [Attrib '\nSAT = on'];
      | end
      | % Update the display
      | set_param(gcb,'AttributesFormatString',Attrib);
      settings: AttributesFormatString=%<MaskType>
      mask TypeOptions Tol: Double Tol | Single Tol | Absolute Zero Tol | User Defined Tol
      mask Callback Tol:
      | %% Make visible or not the Tolerance (update 2nd element of MaskVisibilities)
      | MaskVisibilities = get_param(gcb,'MaskVisibilities');
      | if strcmp(get_param(gcb,'Tol'),'User Defined Tol')
      |     MaskVisibilities{2} = 'on';
      | else
      |     MaskVisibilities{2} = 'off';
      | end
      | set_param(gcb,'MaskVisibilities',MaskVisibilities);
      mask TypeOptions SATOnIntegerOverflow: Switch/SaturateOnIntegerOverflow | While_Iterator/Add/SaturateOnIntegerOverflow
      mask DialogControl SATOnIntegerOverflow Prompt: Saturate on integer overflow
      mask Display:
      | %% Plot the sqrt and display X on the icon
      | plot(-0.1+[.32 3.5/8 4/8 .8],[.5 .25 .75 .75])
      | fprintf('X')
  A_XSquare : Subsystem  Tag=[LIB]  mask(A_XSquare){data_type=Double, prod_OutDataTypeStr=double}
      mask prompts: data_type "Input Data Type"; prod_OutDataTypeStr "Simulink:blkprm_prompts:OUTPUT_UNIFIEDDATATYPE"
      mask help:
      | This block calculates the square of the input 'In'
      |
      | For Integers:
      | 1.  Inputs beyond 0-128 are saturated to 0-128 range.
      | 2.  If the output is beyond than the Output DataType range, then the block saturates to the max value of the output DataType.
      |
      | For Double/Single:
      | 1. Inputs beyond input datatype range are saturated to minimum & maximum of input datatypes.
      |
      | Note:
      | 1. This block will not support for fixed point datatypes with resolution.
      | 2. Input & Output data type of the block has to be chosen by the user
      mask init:
      | %% Block parameters updated based on datatype
      | switch get_param(gcb,'data_type')
      |     case 'Single'
      |         XS_single_Min = -sqrt(realmax('single'));
      |         XS_single_Max = sqrt(realmax('single'));
      |         set_param([gcb '/From1'],'GotoTag','sq_input');
      |         set_param([gcb '/Product'],'SaturateOnIntegerOverflow','off');
      |         set_param([gcb '/Saturation1'],'UpperLimit','XS_single_Max',...
      |             'LowerLimit','XS_single_Min');
      | 
      |     case 'Double'
      |         XS_double_Min = -sqrt(realmax('double'));
      |         XS_double_Max = sqrt(realmax('double'));
      |         set_param([gcb '/From1'],'GotoTag','sq_input');
      |         set_param([gcb '/Product'],'SaturateOnIntegerOverflow','off');
      |         set_param([gcb '/Saturation1'],'UpperLimit','XS_double_Max',...
      |             'LowerLimit','XS_double_Min');
      | 
      |     case 'Integers'
      |         XS_int_Min = 0;
      |         XS_int_Max = 128;
      |         set_param([gcb '/From1'],'GotoTag','In');
      |         set_param([gcb '/Product'],'SaturateOnIntegerOverflow','on');
      |         set_param([gcb '/Saturation1'],'UpperLimit','XS_int_Max',...
      |             'LowerLimit','XS_int_Min');
      | end
      settings: AttributesFormatString=|
      | %<MaskType>
      | In DT = %<data_type>
      | Out DT= %<prod_OutDataTypeStr>
      mask TypeOptions data_type: Single | Double | Integers
      mask TypeOptions prod_OutDataTypeStr: Product/OutDataTypeStr
      mask DialogControl prod_OutDataTypeStr Prompt: Output data type:
      mask Display:
      | %% Display info on the icon
      | fprintf('X^2')

== system Ampere_Library/User_Defined_Libraries/Miscellaneous ==
  note: Saturated resolution signals
  note: Miscellaneous
  A_SigConstrainInvVal : Subsystem  Tag=[LIB]  mask(A_SigConstrainInvVal){Resolution=3, Invalid_Value=-528.4, Max=-253.4, Min=-487.225, tolerance=double tol - eps('double'), user_tol=3}
      mask prompts: Resolution "Data resolution resizing for Resolution Block"; Invalid_Value "Invalid Value"; Max "Maximum Value"; Min "Minimum Value"; tolerance "Tolerance for Invalid Value"; user_tol "User Defined Tolerance"
      mask help:
      | Output will be "Invalid Value" if any of the following is met:
      |     (i) IV + Tol > Res > IV - Tol
      |    (ii) IV - Tol >= Res >=IV + Tol
      |
      |  For remaining cases:
      | This  block will first convert the Input Signal to a resolution specified in the mask parameter and then it will limit the Value between Maximum and Minimum value defined in the mask.
      |
      |  Where,
      |  IV: Invalid Value
      |  Res: Resolution
      |  Tol: Tolerance for Invalid Value
      |
      | Note: This block should be used only with Single and Double Datatypes
      mask init:
      | %% Internal Parameters
      | RF0 = 0;
      | RF1 = 1;
      | RF05 = 0.5;
      | 
      | %% Update the tolerance value
      | switch tolerance
      |     case 1
      |         tol = eps('double');
      |     case 2
      |         tol = eps('single');
      |     case 3
      |         tol = 0;
      |     case 4
      |         tol = user_tol;
      | end
      | 
      | %% Create the infos to display below the block depending of the Mask Options
      | % Always display MaskType / Min / Max
      | Attrib = '%<MaskType>\nMax = %<Max>\nMin = %<Min>';
      | % Conditionnally adding Tolerance
      | if strcmp(get_param(gcb,'tolerance'),'User Defined tol')
      |     Attrib = [Attrib '\nTol = %<user_tol>'];
      | end
      | % Update the display
      | set_param(gcb,'AttributesFormatString',Attrib);
      settings: AttributesFormatString=%<MaskType>\nMax = %<Max>\nMin = %<Min>
      mask TypeOptions tolerance: double tol - eps('double') | single tol - eps('single') | Absolute Zero tol | User Defined tol
      mask Callback tolerance:
      | %% Make visible or not the User Defined Tolerance (update 7th element of MaskVisibilities)
      | MaskVisibilities = get_param(gcb,'MaskVisibilities');
      | if strcmp(get_param(gcb,'tolerance'),'User Defined tol')
      |     MaskVisibilities{6} = 'on';
      | else
      |     MaskVisibilities{6} = 'off';
      | end
      | set_param(gcb,'MaskVisibilities',MaskVisibilities);
      mask Display:
      | %% Display info on the icon
      | fprintf('Resol = %s\nInvalid = %s',get_param(gcb,'Resolution'),get_param(gcb,'Invalid_Value'));
  A_SignalConstraint : Subsystem  Tag=[LIB]  mask(A_SignalConstraint){Resolution=0.01, Max=2.54, Min=-1.27, res_OutDataTypeStr=double}
      mask prompts: Resolution "Signal resolution"; Max "Maximum Value"; Min "Minimum Value"; res_OutDataTypeStr "Simulink:blkprm_prompts:OUTPUT_UNIFIEDDATATYPE"
      mask help: A_SignalConstraint block will first convert the Input Signal to a resolution specified in the mask parameter and then it will limit the Value between Maximum and Minimum value defined in the mask.
      mask init:
      | %% Internal parameters
      | RF0 = 0;
      | RF1 = 1;
      | RF05 = 0.5;
      settings: AttributesFormatString=|
      | %<MaskType>
      | Max = %<Max>
      | Min =  %<Min>
      mask TypeOptions res_OutDataTypeStr: Product1/OutDataTypeStr
      mask DialogControl res_OutDataTypeStr Prompt: Output data type:
      mask Display:
      | %% Display info on the icon
      | fprintf('Resol = %s',get_param(gcb,'Resolution'));
